simulink model "sampleModel1931_2_sub_sub_sub"  (R2023a)
settings: Solver=VariableStepAuto  StartTime=0.0  StopTime=10.0  RelTol=1e-3
libraries: simulink x3, hdlsllib x2
settings Model: Creator=user1  LastModifiedBy=user1
settings OptimizationCC: BlockReduction=off  ConditionallyExecuteInputs=off

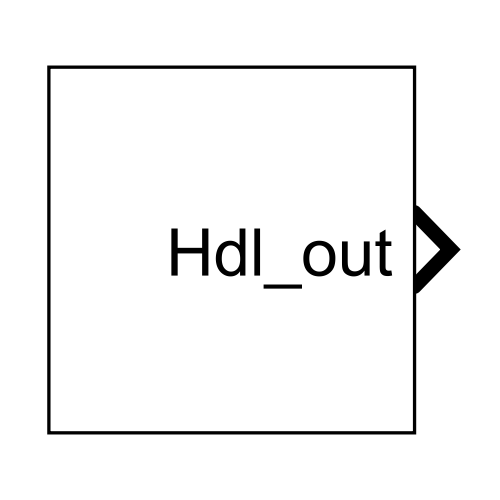
[thumbnail: Simulink's stored preview of the top-level diagram]
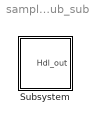
== system sampleModel1931_2_sub_sub_sub ==
  Subsystem : Subsystem

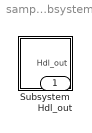
== system sampleModel1931_2_sub_sub_sub/Subsystem ==
  Subsystem : Subsystem
  Hdl_out : Outport  OutDataTypeStr=uint8

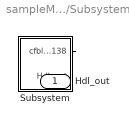
== system sampleModel1931_2_sub_sub_sub/Subsystem/Subsystem ==
  Subsystem : Subsystem
  Hdl_out : Outport  OutDataTypeStr=uint8
  wires:
  Subsystem/1(cfblk138) -> Hdl_out/1

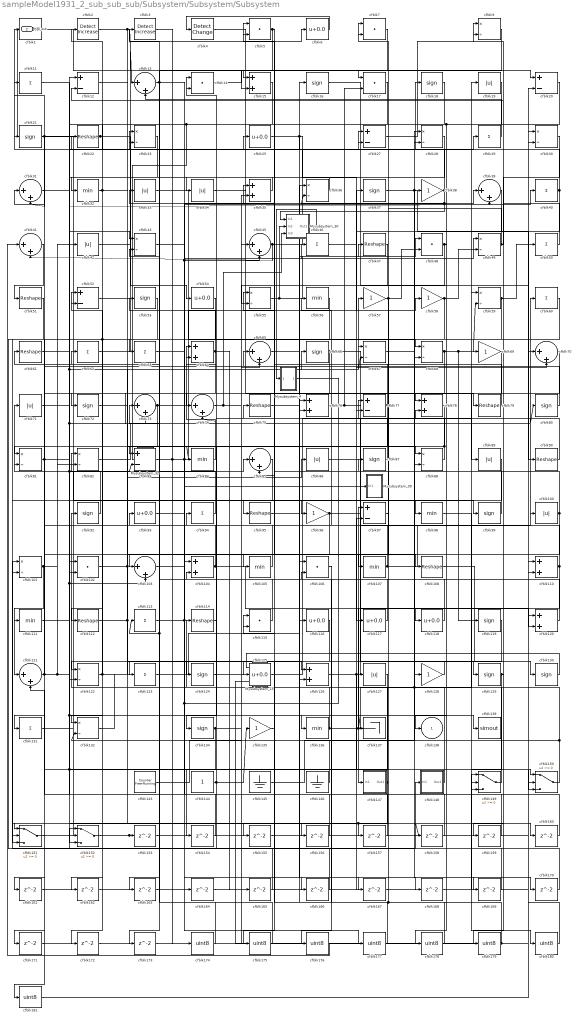
== system sampleModel1931_2_sub_sub_sub/Subsystem/Subsystem/Subsystem ==
  Mysubsystem_15 : Subsystem  TreatAsAtomicUnit=on  RTWFcnName=Mysubsystem_15
      settings: RTWFcnNameOpts=User specified  RTWFileNameOpts=Use function name
  Mysubsystem_30 : Subsystem  TreatAsAtomicUnit=on  RTWFcnName=Mysubsystem_30
      settings: RTWFcnNameOpts=User specified  RTWFileNameOpts=Use function name
  Mysubsystem_32 : Subsystem  TreatAsAtomicUnit=on  RTWFcnName=Mysubsystem_32
      settings: RTWFcnNameOpts=User specified  RTWFileNameOpts=Use function name
  Mysubsystem_39 : Subsystem  TreatAsAtomicUnit=on  RTWFcnName=Mysubsystem_39
      settings: RTWFcnNameOpts=User specified  RTWFileNameOpts=Use function name
  Mysubsystem_7 : Subsystem  TreatAsAtomicUnit=on  RTWFcnName=Mysubsystem_7
      settings: RTWFcnNameOpts=User specified  RTWFileNameOpts=Use function name
  cfblk1 : hdlsllib/Logic and Bit Operations/Compare To Constant  relop=<=  const=3.0  OutDataTypeStr=uint8
  cfblk{19,33..34,42,71,86,89,100,127} (9 alike) : Abs  OutDataTypeStr=uint8  SaturateOnIntegerOverflow=off
  cfblk{9,23,28,30,36,43,49,55,59,67..68,81..82,88,101,122,132} (17 alike) : Product  Inputs=*/  OutDataTypeStr=uint8  RndMeth=Zero  SaturateOnIntegerOverflow=on
  cfblk{5,7,14,17,48,102,106,115} (8 alike) : DotProduct  OutDataTypeStr=uint8
  cfblk{13,31,39,41,45,65,70,73..74,85,103,121} (12 alike) : Sum  Inputs=|++  OutDataTypeStr=uint8
  cfblk{15,35,64,76,78,104,110,120,126} (9 alike) : Sum  OutDataTypeStr=uint8
  cfblk{32,56,84,98,105,107,111,136} (8 alike) : MinMax  OutDataTypeStr=uint8
  cfblk{22,47,51,61,75,79,90,95,108,112,114} (11 alike) : Reshape
  cfblk{11,29,40,46,50,60,62..63,94,113,123,131} (12 alike) : Sum  Inputs=+  OutDataTypeStr=uint8
  cfblk{6,25,54,93,116..118,125} (8 alike) : Bias  Bias=0.0  SaturateOnIntegerOverflow=off
  cfblk{16,18,21,37,53,66,72,80,87,92,99,119,124,129..130,134} (16 alike) : Signum
  cfblk{12,20,27,52,77,83,97} (7 alike) : Sum  Inputs=+-  OutDataTypeStr=uint8
  cfblk{38,57..58,69,96,128,135} (7 alike) : Gain  OutDataTypeStr=uint8
  cfblk137 : Terminator
  cfblk139 : ToWorkspace  VariableName=simout  SaveFormat=Timeseries  SampleTime=-1
  cfblk143 : hdlsllib/Sources/Counter Free-Running  NumBits=16  tsamp=-1
  cfblk144 : Constant  OutDataTypeStr=uint8  SampleTime=-1
  cfblk145 : Ground
  cfblk146 : Ground
  cfblk147 : Subsystem
      settings: LibrarySourceBlock=|
      | hdlsllib/Ports &
      | Subsystems/Subsystem
  cfblk148 : Subsystem
      settings: LibrarySourceBlock=|
      | hdlsllib/Ports &
      | Subsystems/Subsystem
  cfblk{149..152} (4 alike) : Switch  OutDataTypeStr=uint8  SaturateOnIntegerOverflow=off  InputSameDT=off
  cfblk{153..173} (21 alike) : Delay  SampleTime=1
  cfblk{174..181} (8 alike) : DataTypeConversion  OutDataTypeStr=uint8  SaturateOnIntegerOverflow=off  RndMeth=Floor
  cfblk2 : simulink/Logic and Bit Operations/Detect Increase  vinit=0.0  OutDataTypeStr=uint8
      settings: LibrarySourceBlock=|
      | hdlsllib/Logic and Bit
      | Operations/Detect
      | Increase
  cfblk3 : simulink/Logic and Bit Operations/Detect Increase  vinit=0.0  OutDataTypeStr=uint8
      settings: LibrarySourceBlock=|
      | hdlsllib/Logic and Bit
      | Operations/Detect
      | Increase
  cfblk4 : simulink/Logic and Bit Operations/Detect Change  vinit=0  OutDataTypeStr=uint8
      settings: LibrarySourceBlock=|
      | hdlsllib/Logic and Bit
      | Operations/Detect
      | Change
  cfblk138 : Outport  OutDataTypeStr=uint8  VectorParamsAs1DForOutWhenUnconnected=off
  Hdl_out : Outport  Port=2  OutDataTypeStr=uint8
  wires:
  cfblk151/1 -> cfblk85/1
  cfblk59/1 -> cfblk50/1, cfblk162/1, cfblk161/1
  cfblk15/1 -> cfblk152/3, Mysubsystem_32/1(In1)
  cfblk60/1 -> cfblk68/1
  cfblk17/1 -> cfblk73/2
  cfblk1/1 -> cfblk20/1
  cfblk33/1 -> cfblk68/2
  cfblk134/1 -> cfblk171/1, cfblk139/1
  cfblk108/1 -> cfblk130/1
  cfblk146/1 -> cfblk5/1
  cfblk3/1 -> cfblk174/1
  cfblk4/1 -> cfblk79/1
  cfblk66/1 -> cfblk81/1, cfblk98/1
  cfblk62/1 -> cfblk6/1
  cfblk87/1 -> cfblk77/1
  cfblk94/1 -> cfblk71/1
  cfblk149/1 -> cfblk92/1
  cfblk25/1 -> cfblk168/1, cfblk117/1
  cfblk41/1 -> cfblk51/1
  cfblk40/1 -> cfblk2/1, cfblk78/1
  cfblk119/1 -> cfblk123/1
  cfblk22/1 -> Hdl_out/1, cfblk54/1
  cfblk76/1 -> cfblk17/2, cfblk120/2
  cfblk30/1 -> cfblk179/1
  cfblk31/1 -> cfblk155/1, cfblk103/2
  cfblk38/1 -> cfblk1/1, cfblk36/2, Mysubsystem_30/1(In1)
  cfblk103/1 -> cfblk39/1
  cfblk21/1 -> cfblk31/2, cfblk128/1
  cfblk115/1 -> cfblk61/1
  cfblk75/1 -> cfblk48/1
  cfblk79/1 -> cfblk57/1
  cfblk82/1 -> cfblk59/1
  cfblk34/1 -> cfblk89/1
  cfblk2/1 -> cfblk88/1, cfblk13/1
  cfblk27/1 -> cfblk9/1
  cfblk49/1 -> cfblk27/1, cfblk9/2
  cfblk101/1 -> cfblk82/2, cfblk121/1
  cfblk111/1 -> cfblk83/2, cfblk12/1
  cfblk107/1 -> cfblk56/1, cfblk60/1
  cfblk131/1 -> cfblk136/1
  cfblk5/1 -> cfblk105/1, cfblk15/1
  cfblk80/1 -> cfblk21/1
  cfblk53/1 -> cfblk111/1
  cfblk19/1 -> cfblk103/1
  cfblk39/1 -> cfblk77/2
  cfblk68/1 -> cfblk172/1, cfblk119/1, cfblk59/2
  cfblk86/1 -> cfblk129/1
  cfblk117/1 -> cfblk55/1
  cfblk112/1 -> cfblk66/1, cfblk125/1
  cfblk64/1 -> cfblk165/1, cfblk74/1, cfblk53/1
  cfblk90/1 -> cfblk23/1
  cfblk70/1 -> cfblk138/1
  cfblk118/1 -> cfblk65/1
  cfblk16/1 -> cfblk70/1
  cfblk144/1 -> cfblk74/2, cfblk135/1
  cfblk121/1 -> cfblk11/1, cfblk42/1, cfblk156/1, cfblk150/3
  cfblk124/1 -> cfblk58/1
  cfblk42/1 -> cfblk16/1
  cfblk105/1 -> cfblk62/1
  cfblk89/1 -> cfblk134/1
  cfblk7/1 -> cfblk15/2
  cfblk147/1(Out1) -> cfblk151/3, cfblk14/1
  cfblk125/1 -> cfblk69/1
  cfblk45/1 -> cfblk41/2, cfblk29/1
  cfblk114/1 -> cfblk94/1
  cfblk73/1 -> cfblk152/2, cfblk37/1
  cfblk9/1 -> cfblk63/1
  cfblk29/1 -> cfblk13/2
  cfblk126/1 -> cfblk150/2, cfblk78/2
  cfblk100/1 -> cfblk181/1, cfblk27/2
  cfblk20/1 -> cfblk118/1, cfblk72/1
  cfblk35/1 -> cfblk32/1
  cfblk148/1(Out1) -> cfblk115/1
  cfblk136/1 -> cfblk5/2, cfblk97/1, cfblk19/1, cfblk28/2
  cfblk150/1 -> cfblk132/2, cfblk114/1
  cfblk23/1 -> cfblk102/2
  cfblk129/1 -> cfblk159/1, cfblk149/2
  cfblk37/1 -> cfblk99/1, cfblk90/1
  cfblk61/1 -> cfblk137/1, cfblk158/1, cfblk157/1
  cfblk128/1 -> cfblk122/1
  cfblk57/1 -> cfblk48/2, cfblk107/1
  cfblk152/1 -> cfblk153/1, cfblk110/2
  cfblk81/1 -> cfblk31/1, cfblk80/1, cfblk39/2
  cfblk55/1 -> Mysubsystem_30/2(In2), cfblk47/1
  cfblk51/1 -> cfblk148/1(In1)
  cfblk93/1 -> cfblk40/1
  cfblk71/1 -> cfblk67/2, cfblk25/1
  cfblk97/1 -> cfblk7/1
  cfblk32/1 -> cfblk96/1, cfblk112/1
  cfblk122/1 -> cfblk52/2, cfblk86/1
  cfblk52/1 -> cfblk18/1
  cfblk102/1 -> cfblk67/1, cfblk126/1
  cfblk14/1 -> cfblk17/1
  cfblk99/1 -> cfblk22/1
  cfblk43/1 -> cfblk177/1, cfblk45/2
  cfblk13/1 -> cfblk88/2, cfblk83/1
  cfblk47/1 -> cfblk95/1
  cfblk72/1 -> cfblk108/1
  cfblk120/1 -> cfblk104/2
  cfblk83/1 -> cfblk164/1, cfblk46/1, cfblk28/1
  cfblk84/1 -> cfblk64/1
  cfblk78/1 -> cfblk131/1
  cfblk85/1 -> cfblk101/2
  cfblk48/1 -> cfblk178/1, cfblk55/2
  cfblk28/1 -> cfblk122/2
  cfblk145/1 -> cfblk38/1
  cfblk54/1 -> cfblk151/1
  cfblk92/1 -> cfblk82/1
  cfblk65/1 -> cfblk116/1
  cfblk58/1 -> cfblk49/2, cfblk151/2
  cfblk50/1 -> cfblk12/2
  cfblk123/1 -> cfblk36/1
  cfblk69/1 -> cfblk76/2
  cfblk143/1 -> cfblk45/1
  cfblk113/1 -> cfblk150/1, cfblk35/1
  cfblk96/1 -> cfblk132/1, cfblk100/1
  cfblk36/1 -> cfblk34/1
  cfblk104/1 -> cfblk52/1, cfblk147/1(In1)
  cfblk135/1 -> cfblk115/2
  cfblk6/1 -> cfblk4/1
  cfblk88/1 -> cfblk84/1, cfblk64/2
  cfblk110/1 -> cfblk81/2, cfblk127/1
  cfblk46/1 -> cfblk70/2
  cfblk11/1 -> cfblk43/1
  cfblk74/1 -> cfblk49/1, Mysubsystem_30/3(In3)
  cfblk77/1 -> cfblk33/1, cfblk124/1
  cfblk153/1 -> cfblk65/2
  cfblk127/1 -> cfblk154/1
  cfblk154/1 -> cfblk73/1
  cfblk155/1 -> cfblk76/1
  cfblk156/1 -> cfblk102/1
  cfblk157/1 -> cfblk121/2
  cfblk158/1 -> cfblk43/2
  cfblk159/1 -> cfblk85/2
  cfblk12/1 -> cfblk160/1
  cfblk160/1 -> cfblk104/1
  cfblk161/1 -> cfblk149/1
  cfblk162/1 -> cfblk149/3
  cfblk18/1 -> cfblk163/1
  cfblk163/1 -> cfblk126/2
  cfblk164/1 -> cfblk97/2
  cfblk165/1 -> cfblk101/1
  cfblk63/1 -> cfblk166/1
  cfblk166/1 -> cfblk152/1
  cfblk167/1 -> cfblk7/2
  cfblk168/1 -> cfblk120/1
  cfblk95/1 -> cfblk169/1
  cfblk169/1 -> cfblk23/2
  cfblk67/1 -> cfblk170/1
  cfblk170/1 -> cfblk14/2
  cfblk171/1 -> cfblk20/2
  cfblk172/1 -> cfblk110/1
  cfblk56/1 -> cfblk173/1
  cfblk173/1 -> cfblk35/2
  cfblk174/1 -> cfblk113/1, cfblk93/1
  cfblk116/1 -> cfblk175/1
  cfblk175/1 -> cfblk3/1
  cfblk106/1 -> cfblk176/1
  cfblk176/1 -> cfblk41/1
  cfblk177/1 -> cfblk106/1
  cfblk178/1 -> cfblk106/2
  cfblk179/1 -> cfblk75/1, cfblk87/1, Mysubsystem_15/3(In3)
  cfblk98/1 -> cfblk180/1
  cfblk180/1 -> cfblk30/1
  cfblk181/1 -> cfblk30/2
  Mysubsystem_7/1(Out1) -> cfblk167/1, Mysubsystem_39/1(In1)
  cfblk130/1 -> Mysubsystem_15/1(In1)
  cfblk132/1 -> Mysubsystem_15/2(In2)
  Mysubsystem_30/1(Out1) -> Mysubsystem_7/1(In1)

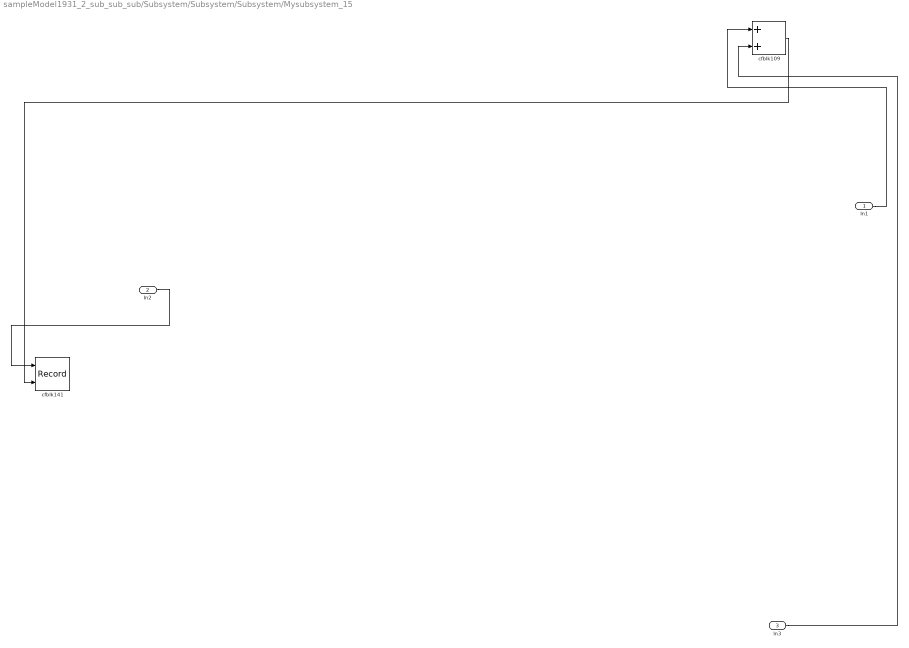
== system sampleModel1931_2_sub_sub_sub/Subsystem/Subsystem/Subsystem/Mysubsystem_15 ==
  In1 : Inport
  In2 : Inport  Port=2
  In3 : Inport  Port=3
  cfblk109 : Sum
  cfblk141 : Record  FileSettingsInternal="{\"entries\":[{\"content\":{\"excelSettings\":{\"content\":{},\"type\":\"Streamout.ExcelSettings\"}},\"type\":\"Streamout.FileSettingStorage\",\"uuid\":\"\"}],\"packageUris\":[\"http:\\/\\/schema.mathworks.com\\/mf0\\/streamout_blocks\\/R2020a\"],\"version\":\"1.0\"}"  Layout=[1 1]  SignalsInternal="{\"entries\":[{\"content\":{},\"type\":\"RecordBlkView.InputSignals\",\"uuid\":\"\"}],\"packageUris\":[\"http:\\/\\/schema.mathworks.com\\/mf0\\/streamout_blocks\\/R2020a\"],\"version\":\"1.0\"}"  VisualizationBindings="{\"xyplotplugin\":{\"info\":[{\"series\":[],\"subplotID\":1}]}}"  CompatibilityTag=XY  st=-1
  wires:
  In3/1 -> cfblk109/2
  cfblk109/1 -> cfblk141/2
  In1/1 -> cfblk109/1
  In2/1 -> cfblk141/1

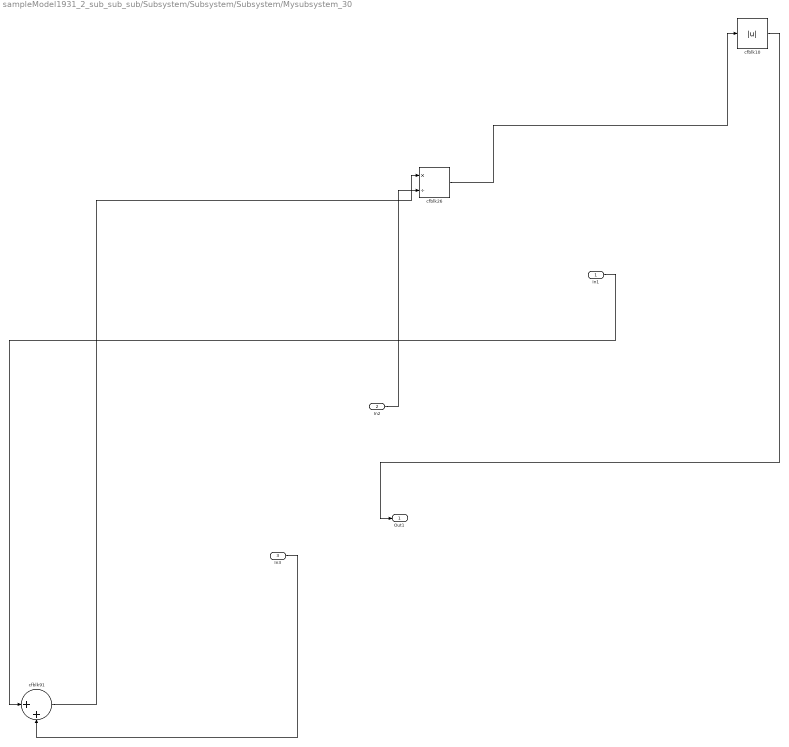
== system sampleModel1931_2_sub_sub_sub/Subsystem/Subsystem/Subsystem/Mysubsystem_30 ==
  In1 : Inport
  In2 : Inport  Port=2
  In3 : Inport  Port=3
  cfblk10 : Abs  SaturateOnIntegerOverflow=off
  cfblk26 : Product  Inputs=*/  RndMeth=Zero  SaturateOnIntegerOverflow=on
  cfblk91 : Sum  Inputs=|++
  Out1 : Outport
  wires:
  In1/1 -> cfblk91/1
  In2/1 -> cfblk26/2
  cfblk91/1 -> cfblk26/1
  cfblk10/1 -> Out1/1
  cfblk26/1 -> cfblk10/1
  In3/1 -> cfblk91/2

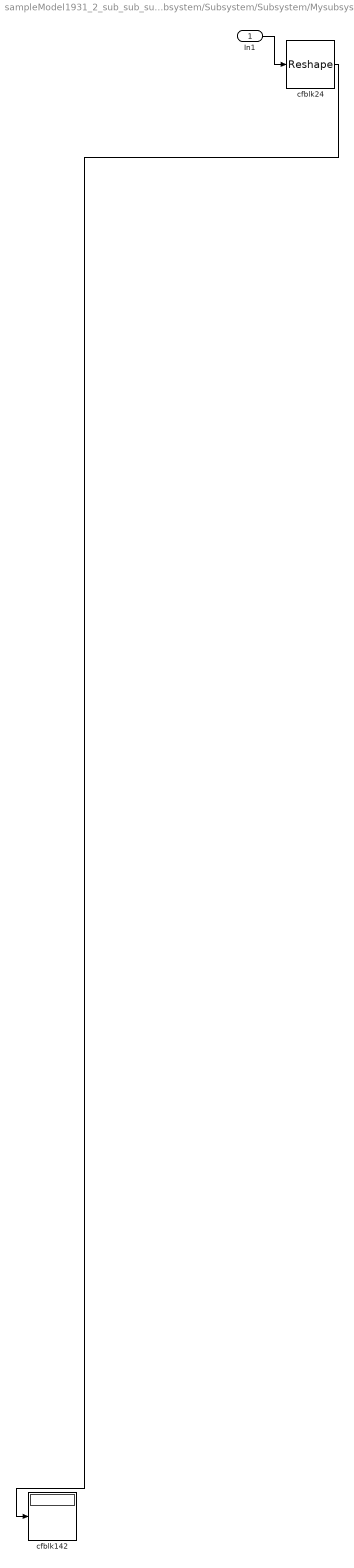
== system sampleModel1931_2_sub_sub_sub/Subsystem/Subsystem/Subsystem/Mysubsystem_32 ==
  In1 : Inport
  cfblk142 : Display
  cfblk24 : Reshape
  wires:
  In1/1 -> cfblk24/1
  cfblk24/1 -> cfblk142/1

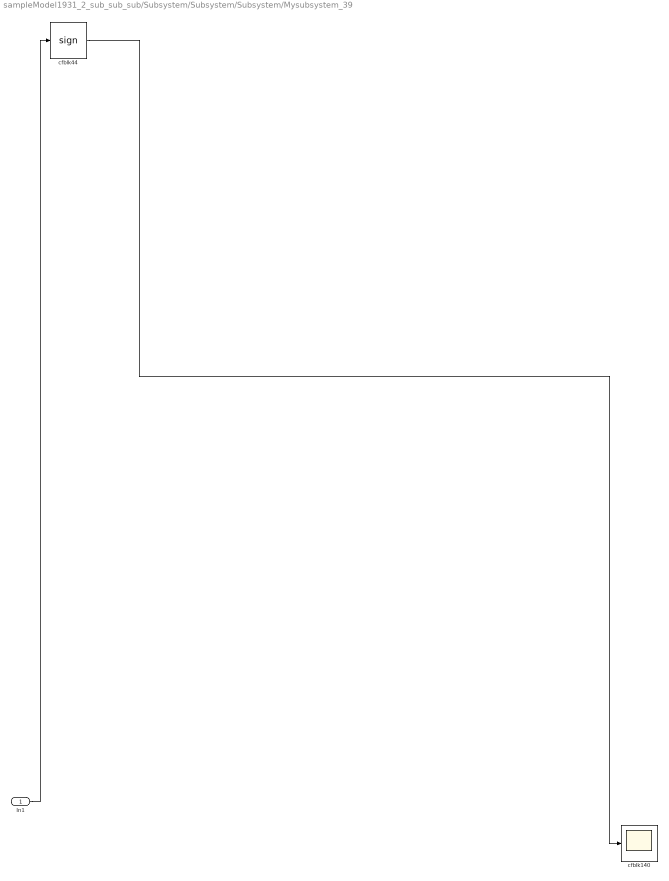
== system sampleModel1931_2_sub_sub_sub/Subsystem/Subsystem/Subsystem/Mysubsystem_39 ==
  In1 : Inport
  cfblk140 : Scope
  cfblk44 : Signum
  wires:
  In1/1 -> cfblk44/1
  cfblk44/1 -> cfblk140/1

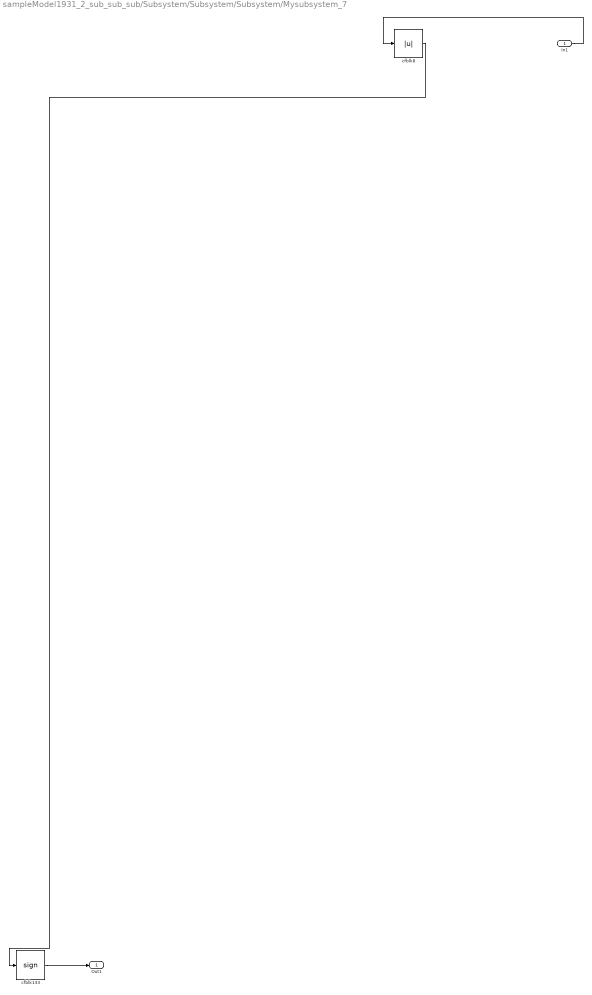
== system sampleModel1931_2_sub_sub_sub/Subsystem/Subsystem/Subsystem/Mysubsystem_7 ==
  In1 : Inport
  cfblk133 : Signum
  cfblk8 : Abs  SaturateOnIntegerOverflow=off
  Out1 : Outport
  wires:
  cfblk133/1 -> Out1/1
  In1/1 -> cfblk8/1
  cfblk8/1 -> cfblk133/1

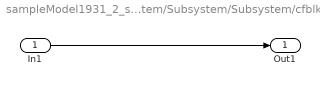
== system sampleModel1931_2_sub_sub_sub/Subsystem/Subsystem/Subsystem/cfblk147 ==
  In1 : Inport
  Out1 : Outport
  wires:
  In1/1 -> Out1/1

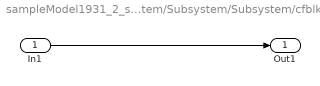
== system sampleModel1931_2_sub_sub_sub/Subsystem/Subsystem/Subsystem/cfblk148 ==
  In1 : Inport
  Out1 : Outport
  wires:
  In1/1 -> Out1/1
